simulink model "QPSK_BER"  (R2026b)
settings: Solver=VariableStepAuto
libraries: commdigbbndpm3 x3, commsink2 x2, dspsigops x1, commrandsrc3 x1, commchan3 x1
settings Model: Creator=Parth  LastModifiedBy=Parth

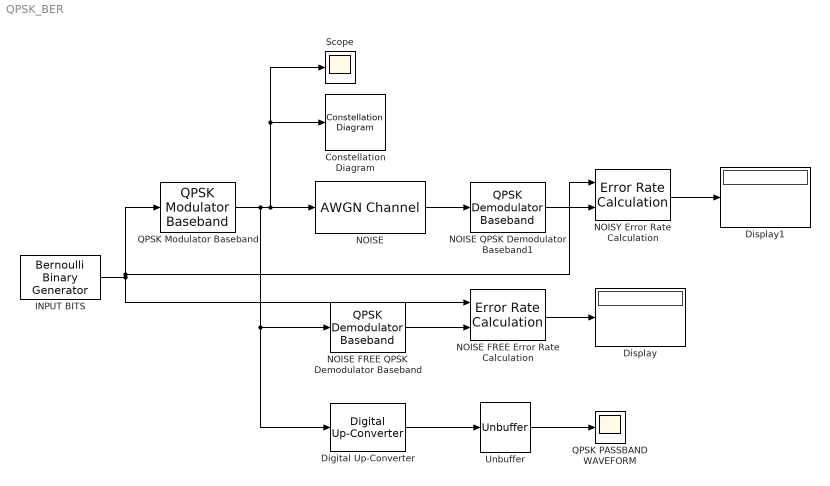
== system QPSK_BER ==
  Constellation Diagram : ConstellationDiagram  WindowPosition=[287.000000,259.000000,600.000000,600.000000,]  Visible=on  ScopeFrameLocation=window  ReferenceConstellation=QPSK  ShowLegend=on
  Digital Up-Converter : dspsigops/Digital Up-Converter  InterpolationFactor=40  MinimumOrderDesign=on  FirstFilterOrder=10  NumCICSections=3  StopbandFrequencySource=Auto  Oscillator=Sine wave  CenterFrequency=500  SecondFilterOrder=12  Bandwidth=0.0133  StopbandFrequency=0.01  PassbandRipple=0.1  StopbandAttenuation=60  NumAccumulatorBits=16  NumQuantizedAccumulatorBits=12  Dither=on  NumDitherBits=4  SampleRateMode=Specify on dialog  SampleRate=100  SimulateUsing=Interpreted execution  outputMin=[]  outputMax=[]
  Display : Display
  Display1 : Display
  INPUT BITS : commrandsrc3/Bernoulli Binary Generator  ProbabilityOfZero=0.5  SeedSource=Parameter  Seed=12345  SampleTime=0.01  SamplesPerFrame=2  OutputDataType=double  SimulateUsing=Interpreted execution
  NOISE : commchan3/AWGN Channel  LegacyMode=off  NoiseMethod="Signal to noise ratio  (Eb/No)"  noiseMode="Signal to noise ratio  (Eb/No)"  EbNo=5  EsNo=5  SNR=5  BitsPerSymbol=2  SignalPower=1  SpecifySymbolPeriod=off  SamplesPerSymbol=1  SymbolPeriod=1  VarianceSource=Parameter  Variance=1  RandomStream=Global stream  Seed=67  SimulateUsing=Code generation
  NOISE FREE Error Rate Calculation : commsink2/Error Rate Calculation  N=0  st_delay=0  cp_mode=Entire frame  subframe=[]  PMode=Port  WsName=ErrorVec  RsMode2=off  stop=off  numErr=100  maxBits=1e6
  NOISE FREE QPSK Demodulator Baseband : commdigbbndpm3/QPSK Demodulator Baseband  OutType=Bit  DecType=Hard decision  VarSource=Dialog  Variance=1  Dec=Gray  Ph=pi/4  outDtype1=Inherit via internal rule  outDtype2=Inherit via internal rule  derotateFactorWordLen=16  derotateFactorDataTypeStr=Inherit: Same word length as input  derotateFactorLastDataTypeStr=Inherit: Same word length as input
  NOISE QPSK Demodulator Baseband1 : commdigbbndpm3/QPSK Demodulator Baseband  OutType=Bit  DecType=Hard decision  VarSource=Dialog  Variance=1  Dec=Gray  Ph=pi/4  outDtype1=Inherit via internal rule  outDtype2=Inherit via internal rule  derotateFactorWordLen=16  derotateFactorDataTypeStr=Inherit: Same word length as input  derotateFactorLastDataTypeStr=Inherit: Same word length as input
  NOISY Error Rate Calculation : commsink2/Error Rate Calculation  N=0  st_delay=0  cp_mode=Entire frame  subframe=[]  PMode=Port  WsName=ErrorVec  RsMode2=off  stop=off  numErr=100  maxBits=1e6
  QPSK Modulator Baseband : commdigbbndpm3/QPSK Modulator Baseband  InType=Bit  Enc=Gray  Ph=pi/4  outDtype=double  outWordLen=16  outUDDataType=sfix(16)  outFracLenMode=Best precision  outFracLen=15  outDataTypeStr=double  outLastDataTypeStr=double
  QPSK PASSBAND WAVEFORM : Scope
      settings: ActiveDisplayYMinimum=-2.1679798240554717  ActiveDisplayYMaximum=1.8825512546719498
  Scope : Scope
      settings: ActiveDisplayYMinimum=-1.0512601393076557  ActiveDisplayYMaximum=0.97400540005605474
  Unbuffer : Unbuffer
  wires:
  Unbuffer/1 -> QPSK PASSBAND WAVEFORM/1
  INPUT BITS/1 -> QPSK Modulator Baseband/1, NOISY Error Rate Calculation/1, NOISE FREE Error Rate Calculation/1
  QPSK Modulator Baseband/1 -> Digital Up-Converter/1, NOISE FREE QPSK Demodulator Baseband/1, Constellation Diagram/1, Scope/1, NOISE/1
  NOISE QPSK Demodulator Baseband1/1 -> NOISY Error Rate Calculation/2
  NOISE/1 -> NOISE QPSK Demodulator Baseband1/1
  NOISE FREE QPSK Demodulator Baseband/1 -> NOISE FREE Error Rate Calculation/2
  Digital Up-Converter/1 -> Unbuffer/1
  NOISE FREE Error Rate Calculation/1 -> Display/1
  NOISY Error Rate Calculation/1 -> Display1/1
